simulink model "ModelUrzadzeniaHamujacegoSamoloty"  (R2024a)
settings: Solver=ode4  StartTime=0.0  StopTime=10.0  FixedStep=0.001  RelTol=1e-3
undefined symbols (not defined in the file): h, k1, k2, m1, m2, m3
settings Model: Creator=adasf  LastModifiedBy=adasf

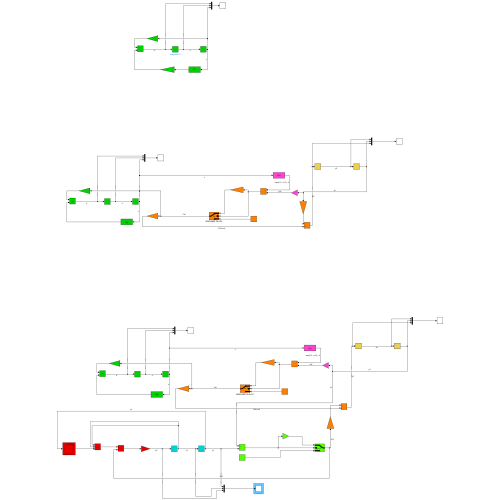
[thumbnail: Simulink's stored preview of the top-level diagram]
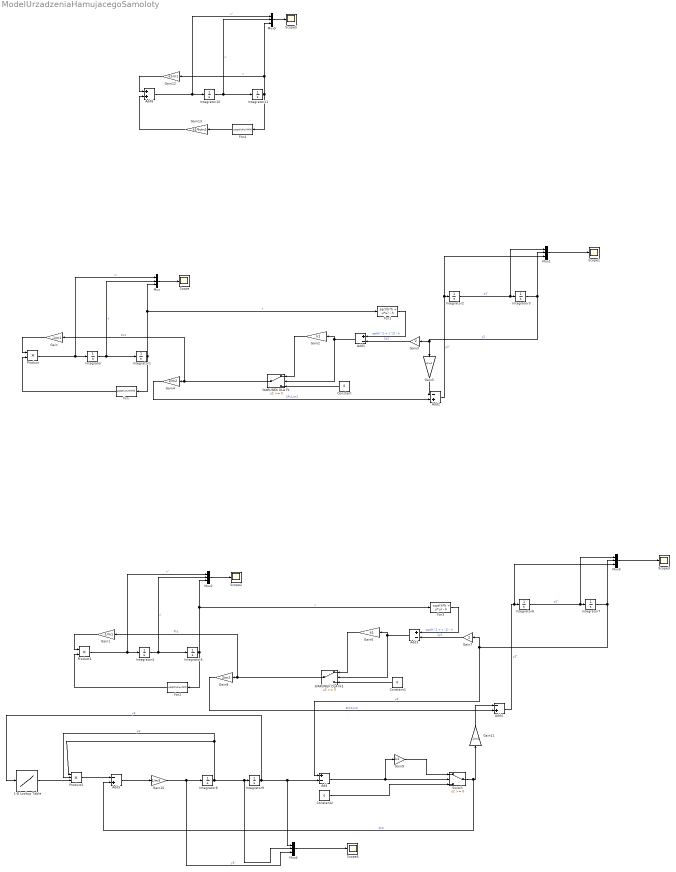
== system ModelUrzadzeniaHamujacegoSamoloty ==
  1-D Lookup Table : Lookup_n-D  NumberOfTableDimensions=1  BreakpointsForDimension1=[0;10;20;30;40;50;60;70;80;90;94;98;102;104;107;120]  Table=[833;400;160;320;520;520;660;830;1070;1600;2100;2800;4100;5000;9000;9000]  InternalRulePriority=Speed  RndMeth=Simplest
  Add : Sum  Inputs=+-
  Add1 : Sum  Inputs=+-
  Add2 : Sum  Inputs=-+
  Add3 : Sum  Inputs=+-
  Add4 : Sum  Inputs=-+
  Add5 : Sum  Inputs=-+
  Add6 : Sum
  Constant : Constant  Value=0
  Constant1 : Constant  Value=0
  Constant2 : Constant  Value=0
  Fcn : Fcn  Expr=u/sqrt(u*u+h*h)
  Fcn1 : Fcn  Expr=sqrt(h*h + u*u) - h
  Fcn2 : Fcn  Expr=u/sqrt(u*u+h*h)
  Fcn3 : Fcn  Expr=sqrt(h*h + u*u) - h
  Fcn4 : Fcn  Expr=u/sqrt(u*u+h*h)
  Gain : Gain  Gain=-1/m1
  Gain1 : Gain  Gain=-1/m1
  Gain10 : Gain  Gain=1/m3
  Gain11 : Gain  Gain=1/m3
  Gain12 : Gain  Gain=-k1/m1
  Gain13 : Gain  Gain=k1*h/m1
  Gain2 : Gain  Gain=k1
  Gain3 : Gain  Gain=2
  Gain4 : Gain  Gain=2/m2
  Gain5 : Gain  Gain=k2/m2
  Gain6 : Gain  Gain=k1
  Gain7 : Gain  Gain=2
  Gain8 : Gain  Gain=2/m2
  Gain9 : Gain  Gain=k2
  Integrator : Integrator  InitialCondition=67
  Integrator{1..3,5..9,11} (9 alike) : Integrator
  Integrator10 : Integrator  InitialCondition=67
  Integrator4 : Integrator  InitialCondition=67
  Mux{,1..5} (6 alike) : Mux  Inputs=3
  Product : Product
  Product1 : Product
  Product2 : Product  Inputs=3
  Scope{,1..5} (6 alike) : Scope
  Switch : Switch  SaturateOnIntegerOverflow=off  InputSameDT=off
  WARUNEK DLA Fk : Switch  SaturateOnIntegerOverflow=off  InputSameDT=off
  WARUNEK DLA Fk1 : Switch  SaturateOnIntegerOverflow=off  InputSameDT=off
  wires:
  Integrator/1 -> Mux/2, Integrator1/1  "x'"
  Product/1 -> Mux/1, Integrator/1  "x\""
  Integrator1/1 -> Mux/3, Fcn1/1, Fcn/1  "x"
  Fcn/1 -> Product/2
  Gain/1 -> Product/1
  Mux/1 -> Scope/1
  Add1/1 -> Gain2/1, WARUNEK DLA Fk/2
  Gain2/1 -> WARUNEK DLA Fk/1
  Constant/1 -> WARUNEK DLA Fk/3
  Fcn1/1 -> Add1/1  "sqrt(h^2 + x^2) - h"
  Gain3/1 -> Add1/2  "2y2"
  Integrator2/1 -> Mux1/1, Integrator3/1  "y2'"
  Integrator3/1 -> Mux1/2, Gain5/1, Gain3/1  "y2"
  WARUNEK DLA Fk/1 -> Gain/1, Gain4/1  "Fk1"
  Gain4/1 -> Add2/2  "2Fk1/m2"
  Gain5/1 -> Add2/1
  Add2/1 -> Mux1/3, Integrator2/1  "y2\""
  Mux1/1 -> Scope1/1
  Fcn2/1 -> Product1/2
  Add4/1 -> Mux3/3, Integrator6/1  "y2\""
  Gain1/1 -> Product1/1
  WARUNEK DLA Fk1/1 -> Gain1/1, Gain8/1  "Fk1"
  Integrator6/1 -> Mux3/1, Integrator7/1  "y2'"
  Gain7/1 -> Add3/2  "2y2"
  Fcn3/1 -> Add3/1  "sqrt(h^2 + x^2) - h"
  Gain6/1 -> WARUNEK DLA Fk1/1
  Constant1/1 -> WARUNEK DLA Fk1/3
  Product1/1 -> Mux2/1, Integrator4/1  "x\""
  Add3/1 -> Gain6/1, WARUNEK DLA Fk1/2
  Mux2/1 -> Scope2/1
  Integrator5/1 -> Mux2/3, Fcn3/1, Fcn2/1  "x"
  Mux3/1 -> Scope3/1
  Integrator7/1 -> Mux3/2, Gain7/1, Add/1  "y2"
  Integrator4/1 -> Mux2/2, Integrator5/1  "x'"
  Gain8/1 -> Add4/2  "2Fk1/m2"
  Gain9/1 -> Switch/1
  Add/1 -> Switch/2, Gain9/1
  Constant2/1 -> Switch/3
  Integrator8/1 -> Product2/2, Product2/1, Mux4/2, Integrator9/1  "y3'"
  Integrator9/1 -> 1-D Lookup Table/1, Mux4/1, Add/2  "y3"
  Gain10/1 -> Mux4/3, Integrator8/1  "y3\""
  Add5/1 -> Gain10/1
  Switch/1 -> Gain11/1, Add5/2  "Fk2"
  Product2/1 -> Add5/1
  1-D Lookup Table/1 -> Product2/3
  Mux4/1 -> Scope4/1
  Gain11/1 -> Add4/1
  Add6/1 -> Mux5/1, Integrator10/1  "x\""
  Gain12/1 -> Add6/1
  Integrator10/1 -> Mux5/2, Integrator11/1  "x'"
  Integrator11/1 -> Gain12/1, Mux5/3, Fcn4/1  "x"
  Fcn4/1 -> Gain13/1
  Mux5/1 -> Scope5/1
  Gain13/1 -> Add6/2
